simulink model "Powertrain_Model"  (R2021a)
settings: Solver=ode45  StartTime=0.0  StopTime=1180  MaxStep=1e-3  RelTol=1e-3
values from neighbouring files (symbols this model uses):
  Area = 1.401    [Powertrain_Model_Script.m]
  cd = 0.679    [Powertrain_Model_Script.m]
  Crf = 0.015    [Powertrain_Model_Script.m]
  Gear_ratio = 4    [Powertrain_Model_Script.m]
  GVM = 270    [Powertrain_Model_Script.m]
  GVW = GVM*g    (= 2648.7)    [Powertrain_Model_Script.m]
  Neff = 0.90    (= 0.9)    [Powertrain_Model_Script.m]
  Rw = 0.2286    [Powertrain_Model_Script.m]
settings Model: PacingRate=631  Creator=SAHIL  LastModifiedBy=Sahil
settings SolverCC: ZeroCrossAlgorithm=Adaptive
settings OptimizationCC: DefaultUnderspecifiedDataType=single
settings DebuggingCC: IgnoredZcDiagnostic=none

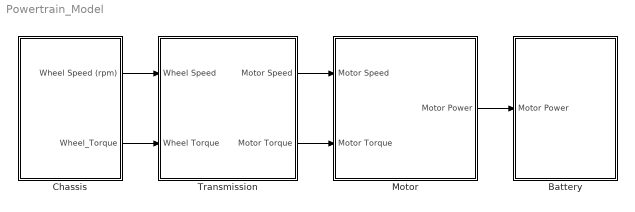
== system Powertrain_Model ==
  Battery : Subsystem
  Chassis : Subsystem
  "Motor " : Subsystem
  "Transmission " : Subsystem
  wires:
  "Motor "/1(Motor Power) -> Battery/1(Motor Power)
  Chassis/1(Wheel Speed (rpm)) -> "Transmission "/1(Wheel Speed)
  Chassis/2(Wheel_Torque) -> "Transmission "/2(Wheel Torque)
  "Transmission "/1(Motor Speed) -> "Motor "/1(Motor Speed)
  "Transmission "/2(Motor Torque) -> "Motor "/2(Motor Torque)

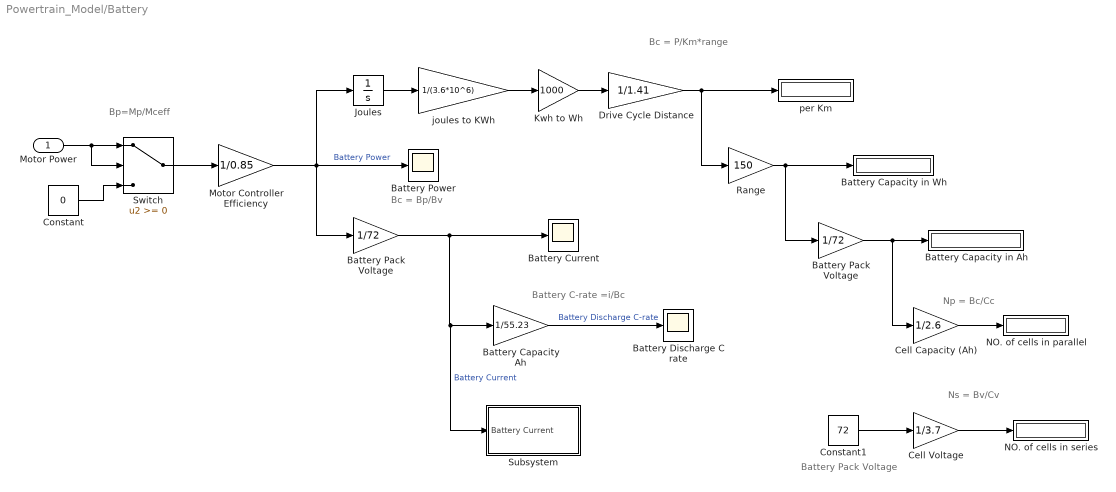
== system Powertrain_Model/Battery ==
  note: Ns = Bv/Cv
  note: Np = Bc/Cc
  note: Bc = P/Km*range
  note: Bc = Bp/Bv
  note: Battery C-rate =i/Bc
  note: Battery Pack Voltage
  note: Bp=Mp/Mceff
  Motor Power : Inport
  Battery Capacity Ah : Gain  Gain=1/55.23
  Battery Capacity in Ah : Display
  Battery Capacity in Wh : Display
  Battery Current : Scope
  Battery Discharge C rate : Scope
  Battery Pack Voltage : Gain  Gain=1/72
  "Battery Pack Voltage " : Gain  Gain=1/72
  Battery Power : Scope
  Cell Capacity (Ah) : Gain  Gain=1/2.6
  "Cell Voltage " : Gain  Gain=1/3.7
  Constant : Constant  Value=0
  Constant1 : Constant  Value=72
  Drive Cycle Distance : Gain  Gain=1/1.41
  "Joules " : Integrator  InitialCondition=1
  Kwh to Wh : Gain  Gain=1000
  Motor Controller Efficiency : Gain  Gain=1/0.85
  NO. of cells in parallel : Display
  NO. of cells in series : Display
  Range : Gain  Gain=150
  Subsystem : Subsystem
  Switch : Switch
  joules to KWh : Gain  Gain=1/(3.6*10^6)
  per Km : Display
  wires:
  Motor Power/1 -> Switch/2, Switch/1
  Constant/1 -> Switch/3
  Switch/1 -> Motor Controller Efficiency/1
  Motor Controller Efficiency/1 -> Battery Power/1, "Battery Pack Voltage "/1, "Joules "/1  "Battery Power"
  joules to KWh/1 -> Kwh to Wh/1
  "Joules "/1 -> joules to KWh/1
  Kwh to Wh/1 -> Drive Cycle Distance/1
  Constant1/1 -> "Cell Voltage "/1
  "Cell Voltage "/1 -> NO. of cells in series/1
  "Battery Pack Voltage "/1 -> Battery Current/1, Subsystem/1(Battery Current), Battery Capacity Ah/1  "Battery Current"
  Battery Capacity Ah/1 -> Battery Discharge C rate/1  "Battery Discharge C-rate"
  Drive Cycle Distance/1 -> per Km/1, Range/1
  Range/1 -> Battery Pack Voltage/1, Battery Capacity in Wh/1
  Battery Pack Voltage/1 -> Battery Capacity in Ah/1, Cell Capacity (Ah)/1
  Cell Capacity (Ah)/1 -> NO. of cells in parallel/1

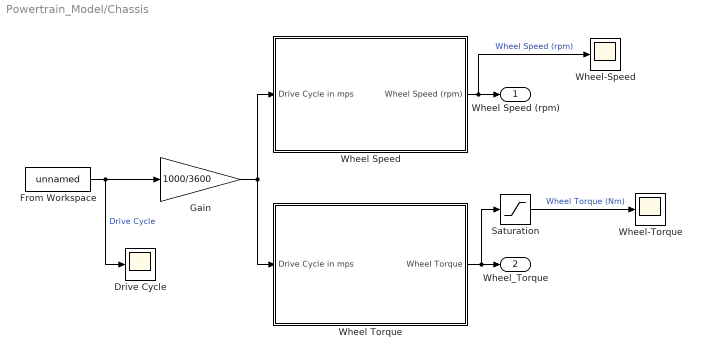
== system Powertrain_Model/Chassis ==
  Drive Cycle : Scope
  From Workspace : FromWorkspace  VariableName=unnamed
  Gain : Gain  Gain=1000/3600
  Saturation : Saturate  UpperLimit=inf  LowerLimit=0
  "Wheel Speed " : Subsystem
  Wheel Torque : Subsystem
  Wheel-Speed : Scope
  Wheel-Torque : Scope
  Wheel Speed (rpm) : Outport
  Wheel_Torque : Outport  Port=2
  wires:
  Gain/1 -> Wheel Torque/1(Drive Cycle in mps), "Wheel Speed "/1(Drive Cycle in mps)
  "Wheel Speed "/1(Wheel Speed (rpm)) -> Wheel-Speed/1, Wheel Speed (rpm)/1  "Wheel Speed (rpm)"
  Wheel Torque/1(Wheel Torque) -> Saturation/1, Wheel_Torque/1
  From Workspace/1 -> Drive Cycle/1, Gain/1  "Drive Cycle"
  Saturation/1 -> Wheel-Torque/1  "Wheel Torque (Nm)"

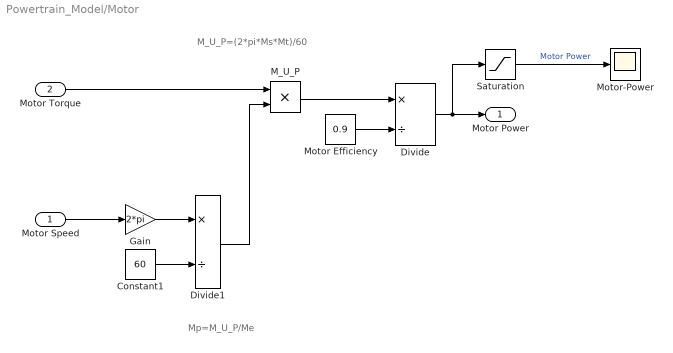
== system Powertrain_Model/Motor  ==
  note: Mp=M_U_P/Me
  note: M_U_P=(2*pi*Ms*Mt)/60
  Motor Speed : Inport
  Motor Torque : Inport  Port=2
  Constant1 : Constant  Value=60
  Divide : Product  Inputs=*/
  Divide1 : Product  Inputs=*/
  Gain : Gain  Gain=2*pi
  M_U_P : Product
  Motor Efficiency : Constant  Value=0.9
  Motor-Power : Scope
  Saturation : Saturate  UpperLimit=inf  LowerLimit=0
  Motor Power : Outport
  wires:
  Motor Speed/1 -> Gain/1
  Gain/1 -> Divide1/1
  Constant1/1 -> Divide1/2
  Divide1/1 -> M_U_P/2
  Motor Efficiency/1 -> Divide/2
  M_U_P/1 -> Divide/1
  Motor Torque/1 -> M_U_P/1
  Divide/1 -> Saturation/1, Motor Power/1
  Saturation/1 -> Motor-Power/1  "Motor Power"

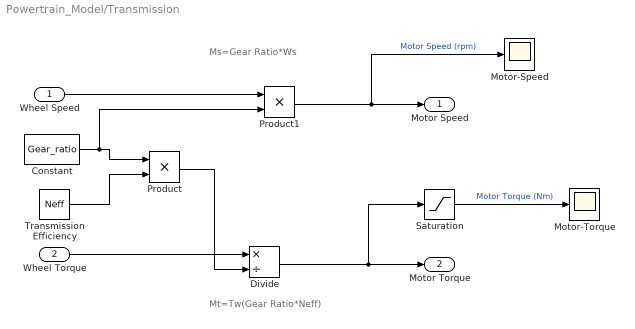
== system Powertrain_Model/Transmission  ==
  note: Mt=Tw(Gear Ratio*Neff)
  note: Ms=Gear Ratio*Ws
  Wheel Speed : Inport
  Wheel Torque : Inport  Port=2
  Constant : Constant  Value=Gear_ratio
  Divide : Product  Inputs=*/
  Motor-Speed : Scope
  Motor-Torque : Scope
  Product : Product
  Product1 : Product
  Saturation : Saturate  UpperLimit=inf  LowerLimit=0
  Transmission Efficiency : Constant  Value=Neff
  Motor Speed : Outport
  Motor Torque : Outport  Port=2
  wires:
  Wheel Torque/1 -> Divide/1
  Product/1 -> Divide/2
  Constant/1 -> Product1/2, Product/1
  Transmission Efficiency/1 -> Product/2
  Wheel Speed/1 -> Product1/1
  Product1/1 -> Motor-Speed/1, Motor Speed/1  "Motor Speed (rpm)"
  Divide/1 -> Saturation/1, Motor Torque/1
  Saturation/1 -> Motor-Torque/1  "Motor Torque (Nm)"

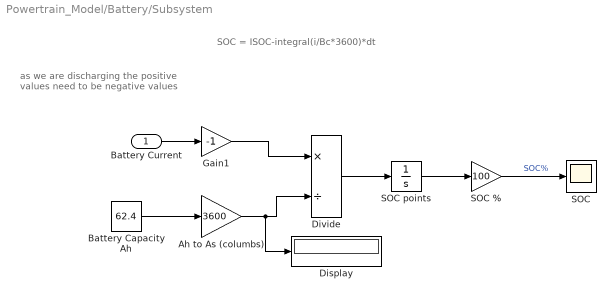
== system Powertrain_Model/Battery/Subsystem ==
  note: as we are discharging the positive values need to be negative values
  note: SOC = ISOC-integral(i/Bc*3600)*dt
  Battery Current : Inport
  Ah to As (columbs) : Gain  Gain=3600
  Battery Capacity Ah : Constant  Value=62.4
  Display : Display
      settings: Format=decimal (Stored Integer)
  Divide : Product  Inputs=*/
  Gain1 : Gain  Gain=-1
  SOC : Scope
  SOC % : Gain  Gain=100
  SOC points : Integrator  InitialCondition=1
  wires:
  Battery Capacity Ah/1 -> Ah to As (columbs)/1
  Battery Current/1 -> Gain1/1
  Gain1/1 -> Divide/1
  Ah to As (columbs)/1 -> Display/1, Divide/2
  SOC points/1 -> SOC %/1
  Divide/1 -> SOC points/1
  SOC %/1 -> SOC/1  "SOC%"

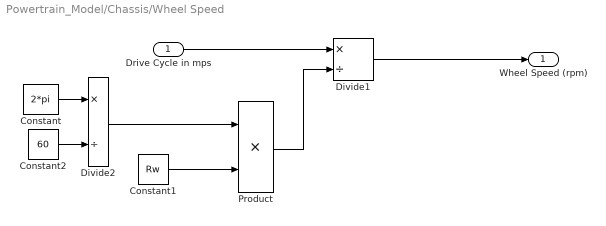
== system Powertrain_Model/Chassis/Wheel Speed  ==
  Drive Cycle in mps : Inport
  Constant : Constant  Value=2*pi
  Constant1 : Constant  Value=Rw
  Constant2 : Constant  Value=60
  Divide1 : Product  Inputs=*/
  Divide2 : Product  Inputs=*/
  Product : Product
  Wheel Speed (rpm) : Outport
  wires:
  Drive Cycle in mps/1 -> Divide1/1
  Divide1/1 -> Wheel Speed (rpm)/1
  Product/1 -> Divide1/2
  Constant1/1 -> Product/2
  Constant/1 -> Divide2/1
  Constant2/1 -> Divide2/2
  Divide2/1 -> Product/1

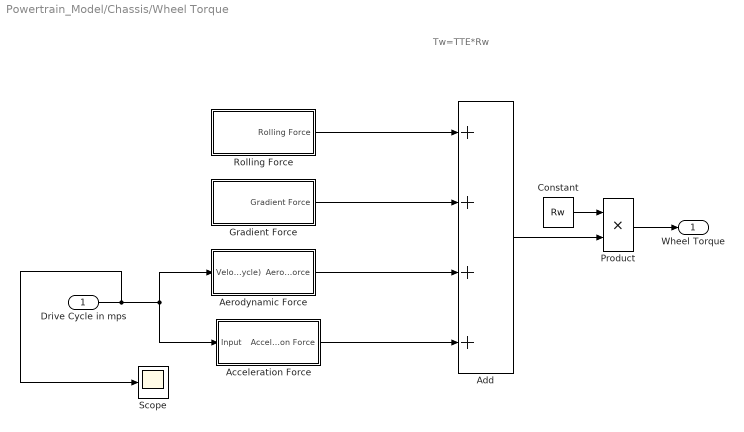
== system Powertrain_Model/Chassis/Wheel Torque ==
  note: Tw=TTE*Rw
  Drive Cycle in mps : Inport
  Acceleration Force : Subsystem
  Add : Sum  Inputs=++++
  Aerodynamic Force : Subsystem
  Constant : Constant  Value=Rw
  Gradient Force : Subsystem  TreatAsAtomicUnit=on
  Product : Product
  Rolling Force : Subsystem  TreatAsAtomicUnit=on
  Scope : Scope
  Wheel Torque : Outport
  wires:
  Aerodynamic Force/1(Aerodynamic Force) -> Add/3
  Acceleration Force/1(Acceleration Force) -> Add/4
  Product/1 -> Wheel Torque/1
  Constant/1 -> Product/1
  Add/1 -> Product/2
  Drive Cycle in mps/1 -> Scope/1, Acceleration Force/1(Input), Aerodynamic Force/1(Velocity (drive cycle))
  Rolling Force/1(Rolling Force) -> Add/1
  Gradient Force/1(Gradient Force) -> Add/2

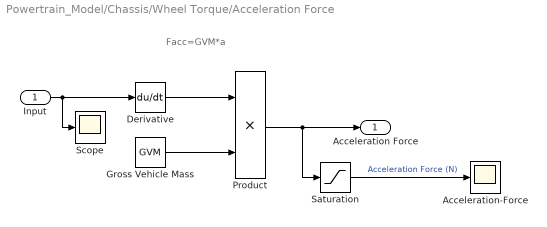
== system Powertrain_Model/Chassis/Wheel Torque/Acceleration Force ==
  note: Facc=GVM*a
  Input : Inport
  Acceleration-Force : Scope
  Derivative : Derivative  CoefficientInTFapproximation=0
  Gross Vehicle Mass : Constant  Value=GVM
  Product : Product
  Saturation : Saturate  UpperLimit=inf  LowerLimit=0
  Scope : Scope
  Acceleration Force : Outport
  wires:
  Gross Vehicle Mass/1 -> Product/2
  Product/1 -> Saturation/1, Acceleration Force/1
  Derivative/1 -> Product/1
  Input/1 -> Scope/1, Derivative/1
  Saturation/1 -> Acceleration-Force/1  "Acceleration Force (N)"

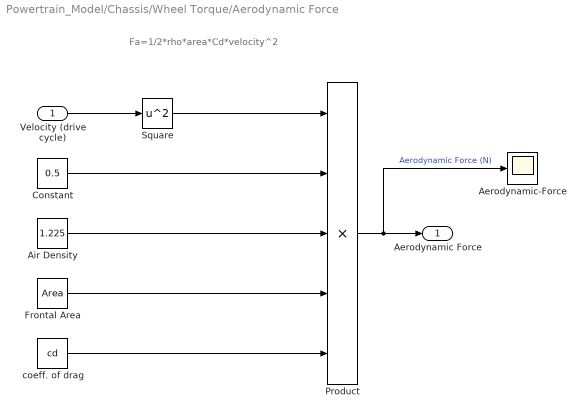
== system Powertrain_Model/Chassis/Wheel Torque/Aerodynamic Force ==
  note: Fa=1/2*rho*area*Cd*velocity^2
  Velocity (drive cycle) : Inport
  Aerodynamic-Force : Scope
  Air Density : Constant  Value=1.225
  Constant : Constant  Value=0.5
  Frontal Area : Constant  Value=Area
  Product : Product  Inputs=5
  Square : Math  Operator=square  SaturateOnIntegerOverflow=on
  coeff. of drag : Constant  Value=cd
  Aerodynamic Force : Outport
  wires:
  Velocity (drive cycle)/1 -> Square/1
  Square/1 -> Product/1
  coeff. of drag/1 -> Product/5
  Frontal Area/1 -> Product/4
  Air Density/1 -> Product/3
  Constant/1 -> Product/2
  Product/1 -> Aerodynamic-Force/1, Aerodynamic Force/1  "Aerodynamic Force (N)"

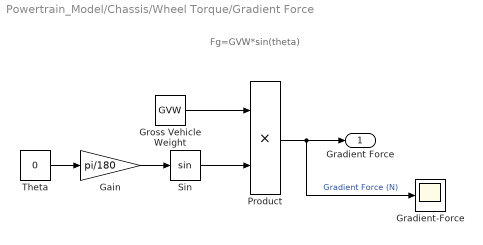
== system Powertrain_Model/Chassis/Wheel Torque/Gradient Force ==
  note: Fg=GVW*sin(theta)
  Gain : Gain  Gain=pi/180
  Gradient-Force : Scope
  Gross Vehicle Weight : Constant  Value=GVW
  Product : Product
  Sin : Trigonometry
  Theta : Constant  Value=0
  Gradient Force : Outport
  wires:
  Product/1 -> Gradient-Force/1, Gradient Force/1  "Gradient Force (N)"
  Gross Vehicle Weight/1 -> Product/1
  Sin/1 -> Product/2
  Gain/1 -> Sin/1
  Theta/1 -> Gain/1

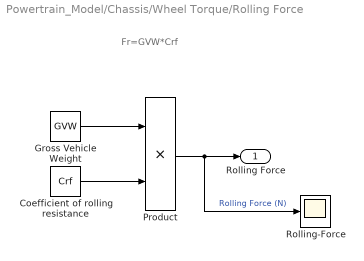
== system Powertrain_Model/Chassis/Wheel Torque/Rolling Force ==
  note: Fr=GVW*Crf
  Coefficient of rolling resistance : Constant  Value=Crf
  Gross Vehicle Weight : Constant  Value=GVW
  Product : Product
  Rolling-Force : Scope
  Rolling Force : Outport
  wires:
  Gross Vehicle Weight/1 -> Product/1
  Coefficient of rolling resistance/1 -> Product/2
  Product/1 -> Rolling-Force/1, Rolling Force/1  "Rolling Force (N)"
